simulink model "Organic_AH2"  (R2019b)
settings: Solver=VariableStepAuto  StartTime=0.0  StopTime=t_sim  RelTol=1e-3
InitFcn:
  | clc
  | %clear
  | Ci = 10e-12;
  | t_sim = 40;
  | Vds_max = 10;
  | Vds_min = 0;
  | slope = (Vds_max-Vds_min)/t_sim;
values from neighbouring files (symbols this model uses):
  l = 100e-6    (= 0.0001)    [oAH_main1.m]    (also in oAH_main2.m; oAH_main3.m; oAH_main4.m)
libraries: fl_lib x12, nesl_utility x4
settings Model: Creator=M.J. Mir  LastModifiedBy=yeeyoung
settings SFSimCC: CustomCodeUndefinedFunction=UseInterfaceOnly
settings SimscapeCC: SimscapeNormalizeSystem=off

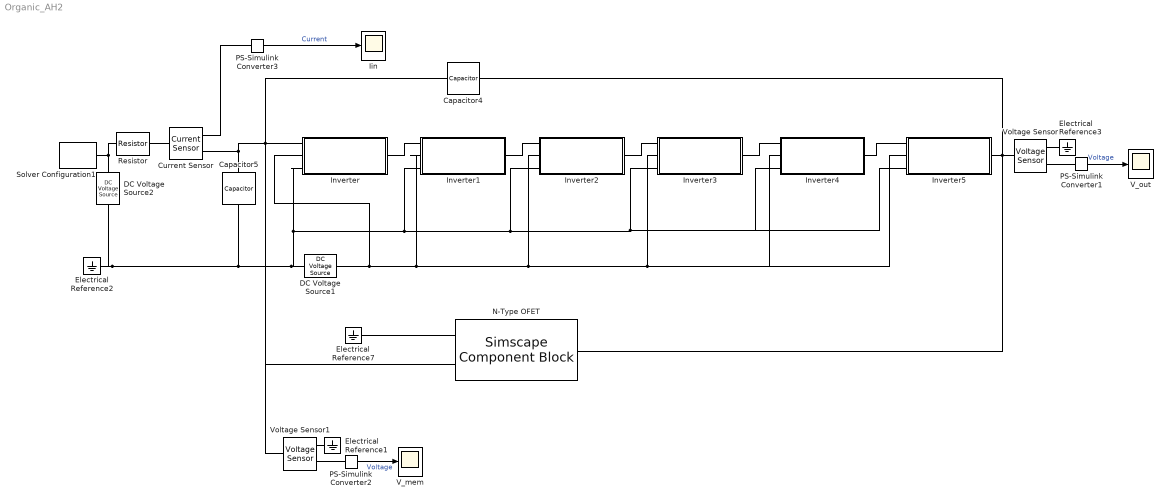
== system Organic_AH2 ==
  Capacitor4 : fl_lib/Electrical/Electrical Elements/Capacitor  c=Cfb nF  r=1e-6 Ohm  g=0 1/Ohm  i_specify=off  i_priority=None  i=0 A  i_nominal_specify=off  i_nominal_unit=A  i_nominal_value=1  v_specify=off  v_priority=None  v=0 V  v_nominal_specify=off  v_nominal_unit=V  v_nominal_value=1  vc_specify=off  vc_priority=High  vc=0 V  vc_nominal_specify=off  vc_nominal_unit=V  vc_nominal_value=1
  Capacitor5 : fl_lib/Electrical/Electrical Elements/Capacitor  c=Cmem nF  r=1e-6 Ohm  g=0 1/Ohm  i_specify=off  i_priority=None  i=0 A  i_nominal_specify=off  i_nominal_unit=A  i_nominal_value=1  v_specify=off  v_priority=None  v=0 V  v_nominal_specify=off  v_nominal_unit=V  v_nominal_value=1  vc_specify=off  vc_priority=High  vc=0 V  vc_nominal_specify=off  vc_nominal_unit=V  vc_nominal_value=1
  Current Sensor : fl_lib/Electrical/Electrical Sensors/Current Sensor
  DC Voltage Source1 : fl_lib/Electrical/Electrical Sources/DC Voltage Source  v0=Vdd V
  DC Voltage Source2 : fl_lib/Electrical/Electrical Sources/DC Voltage Source  v0=Vin V
  Electrical Reference{1..3,7} (4 alike) : fl_lib/Electrical/Electrical Elements/Electrical Reference
  Iin : Scope
  Inverter : Subsystem
  Inverter1 : Subsystem
  Inverter2 : Subsystem
  Inverter3 : Subsystem
  Inverter4 : Subsystem
  Inverter5 : Subsystem
  N-Type OFET : SimscapeComponentBlock  SourceFile=N_Marinov_OFET  ComponentPath=N_Marinov_OFET  ComponentVariants=N_Marinov_OFET  ComponentVariantNames=N_Marinov_OFET  ClassName=N_Marinov_OFET  SchemaVersion=1  Gamma=gama_n  Lambda=landa_n  Vbb=Vbb_n  Vss=Vss_n  Mu0=mu0_n  Vt=Vt_n V  Cox=ci  W=W_n  L=l  i_specify=off  i_priority=None  i=0 A  i_nominal_specify=off  i_nominal_unit=A  i_nominal_value=1  Vgs_specify=off  Vgs_priority=None  Vgs=0 V  Vgs_nominal_specify=off  Vgs_nominal_unit=V  Vgs_nominal_value=1  Vds_specify=off  Vds_priority=None  Vds=0 V  Vds_nominal_specify=off  Vds_nominal_unit=V  Vds_nominal_value=1
      settings: CopyFcn=simscape.engine.sli.internal.componentblockcallback(gcbh,'COPY')  PreCopyFcn=simscape.engine.sli.internal.componentblockcallback(gcbh,'PRECOPY')  PreDeleteFcn=simscape.engine.sli.internal.componentblockcallback(gcbh,'PREDELETE')  InternalSimscapePortConfiguration="{\"Bottom\":[],\"Left\":[{\"id\":\"g\",\"label\":\"Gate\",\"type\":\"foundation.electrical.electrical\"}],\"Right\":[{\"id\":\"d\",\"label\":\"Drain\",\"type\":\"foundation.electrical.electrical\"},{\"id\":\"s\",\"label\":\"Source\",\"type\":\"foundation.electrical.electrical\"}],\"Top\":[]}"
      mask Type: Marinov OFET
  PS-Simulink Converter1 : nesl_utility/PS-Simulink Converter  PhysicalDomain=network_engine_domain  SubClassName=ps_output  LeftPortType=input  RightPortType=output  PseudoPeriodic=off  Frequencies=[]  Unit=1  AffineConversion=off
  PS-Simulink Converter2 : nesl_utility/PS-Simulink Converter  PhysicalDomain=network_engine_domain  SubClassName=ps_output  LeftPortType=input  RightPortType=output  PseudoPeriodic=off  Frequencies=[]  Unit=1  AffineConversion=off
  PS-Simulink Converter3 : nesl_utility/PS-Simulink Converter  PhysicalDomain=network_engine_domain  SubClassName=ps_output  LeftPortType=input  RightPortType=output  PseudoPeriodic=off  Frequencies=[]  Unit=1  AffineConversion=off
  Resistor : fl_lib/Electrical/Electrical Elements/Resistor  R=10 MOhm  i_specify=off  i_priority=None  i=0 A  i_nominal_specify=off  i_nominal_unit=A  i_nominal_value=1  v_specify=off  v_priority=None  v=0 V  v_nominal_specify=off  v_nominal_unit=V  v_nominal_value=1
  Solver Configuration1 : nesl_utility/Solver Configuration  PhysicalDomain=network_engine_domain  SubClassName=solver  LeftPortType=input  RightPortType=generic  Tones=[]  Harmonics=[]  SimulateNoise=off  Profile=off  UseLocalSampling=off  EnableSwitchedLinearOptims=on  FrequencyDomain=off  UseCCode=off  RelTol=0.001  AbsTol=1e-06  MinStep=1e-09  ToWorkspace=off  RevertToSquareIcSolve=off  NumHomotopyIterations=100  PhasorMode=off  PhasorModeNumHarmonics=1  DoDC=off  ResidualTolerance=1e-09  UseLocalSolver=off  LocalSolverChoice=NE_BACKWARD_EULER_ADVANCER  LocalSolverSampleTime=0.001  DoFixedCost=off  MaxNonlinIter=3  MaxModeIter=2  LinearAlgebra=auto  EquationFormulation=NE_TIME_EF  DelaysMemoryBudget=1024  AutomaticFiltering=off  FilteringTimeConstant=0.001  PartitionStorageMethod=AS_NEEDED  PartitionMemoryBudget=1024  PartitionMethod=ROBUST
  V_mem : Scope
  V_out : Scope
  Voltage Sensor : fl_lib/Electrical/Electrical Sensors/Voltage Sensor
  Voltage Sensor1 : fl_lib/Electrical/Electrical Sensors/Voltage Sensor
  wires:
  PS-Simulink Converter1/1 -> V_out/1  "Voltage"
  PS-Simulink Converter2/1 -> V_mem/1  "Voltage"
  PS-Simulink Converter3/1 -> Iin/1  "Current"
  connections:
  Electrical Reference2/LConn1 -- DC Voltage Source2/RConn1 -- Capacitor5/RConn1 -- Inverter1/LConn3 -- Inverter5/LConn3 -- Inverter4/LConn3 -- Inverter3/LConn3 -- Inverter2/LConn3 -- Inverter/LConn3 -- DC Voltage Source1/RConn1
  Voltage Sensor/RConn1 -- PS-Simulink Converter1/LConn1
  Voltage Sensor/RConn2 -- Electrical Reference3/LConn1
  Capacitor5/LConn1 -- Current Sensor/RConn2 -- N-Type OFET/RConn1 -- Voltage Sensor1/LConn1 -- Inverter/LConn1 -- Capacitor4/LConn1
  DC Voltage Source2/LConn1 -- Solver Configuration1/RConn1 -- Resistor/LConn1
  Inverter1/LConn1 -- Inverter/RConn1
  Inverter1/RConn1 -- Inverter2/LConn1
  Inverter2/RConn1 -- Inverter3/LConn1
  Inverter4/LConn2 -- Inverter5/LConn2 -- Inverter3/LConn2 -- Inverter2/LConn2 -- Inverter1/LConn2 -- Inverter/LConn2 -- DC Voltage Source1/LConn1
  Voltage Sensor1/RConn2 -- Electrical Reference1/LConn1
  Voltage Sensor1/RConn1 -- PS-Simulink Converter2/LConn1
  N-Type OFET/RConn2 -- Electrical Reference7/LConn1
  Inverter5/RConn1 -- Voltage Sensor/LConn1 -- N-Type OFET/LConn1 -- Capacitor4/RConn1
  Inverter4/LConn1 -- Inverter3/RConn1
  Inverter5/LConn1 -- Inverter4/RConn1
  Resistor/RConn1 -- Current Sensor/LConn1
  PS-Simulink Converter3/LConn1 -- Current Sensor/RConn1

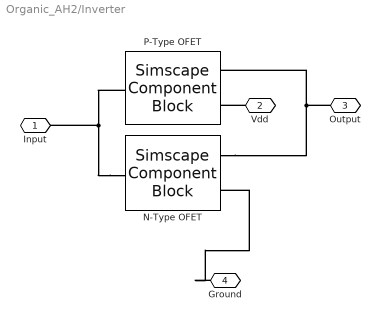
== system Organic_AH2/Inverter ==
  N-Type OFET : SimscapeComponentBlock  SourceFile=N_Marinov_OFET  ComponentPath=N_Marinov_OFET  ComponentVariants=N_Marinov_OFET  ComponentVariantNames=N_Marinov_OFET  ClassName=N_Marinov_OFET  SchemaVersion=1  Gamma=gama_n  Lambda=landa_n  Vbb=Vbb_n  Vss=Vss_n  Mu0=mu0_n  Vt=Vt_n V  Cox=ci  W=W_n  L=l  i_specify=off  i_priority=None  i=0 A  i_nominal_specify=off  i_nominal_unit=A  i_nominal_value=1  Vgs_specify=off  Vgs_priority=None  Vgs=0 V  Vgs_nominal_specify=off  Vgs_nominal_unit=V  Vgs_nominal_value=1  Vds_specify=off  Vds_priority=None  Vds=0 V  Vds_nominal_specify=off  Vds_nominal_unit=V  Vds_nominal_value=1
      settings: CopyFcn=simscape.engine.sli.internal.componentblockcallback(gcbh,'COPY')  PreCopyFcn=simscape.engine.sli.internal.componentblockcallback(gcbh,'PRECOPY')  PreDeleteFcn=simscape.engine.sli.internal.componentblockcallback(gcbh,'PREDELETE')  InternalSimscapePortConfiguration="{\"Bottom\":[],\"Left\":[{\"id\":\"g\",\"label\":\"Gate\",\"type\":\"foundation.electrical.electrical\"}],\"Right\":[{\"id\":\"d\",\"label\":\"Drain\",\"type\":\"foundation.electrical.electrical\"},{\"id\":\"s\",\"label\":\"Source\",\"type\":\"foundation.electrical.electrical\"}],\"Top\":[]}"
      mask Type: Marinov OFET
  P-Type OFET : SimscapeComponentBlock  SourceFile=P_Marinov_OFET  ComponentPath=P_Marinov_OFET  ComponentVariants=P_Marinov_OFET  ComponentVariantNames=P_Marinov_OFET  ClassName=P_Marinov_OFET  SchemaVersion=1  Gamma=gama_p  Lambda=landa_p  Vbb=Vbb_p  Vss=Vss_p  Mu0=mu0_p  Vt=Vt_p V  Cox=ci  W=W_p  L=l  i_specify=off  i_priority=None  i=0 A  i_nominal_specify=off  i_nominal_unit=A  i_nominal_value=1  Vsg_specify=off  Vsg_priority=None  Vsg=0 V  Vsg_nominal_specify=off  Vsg_nominal_unit=V  Vsg_nominal_value=1  Vsd_specify=off  Vsd_priority=None  Vsd=0 V  Vsd_nominal_specify=off  Vsd_nominal_unit=V  Vsd_nominal_value=1
      settings: CopyFcn=simscape.engine.sli.internal.componentblockcallback(gcbh,'COPY')  PreCopyFcn=simscape.engine.sli.internal.componentblockcallback(gcbh,'PRECOPY')  PreDeleteFcn=simscape.engine.sli.internal.componentblockcallback(gcbh,'PREDELETE')  InternalSimscapePortConfiguration="{\"Bottom\":[],\"Left\":[{\"id\":\"g\",\"label\":\"Gate\",\"type\":\"foundation.electrical.electrical\"}],\"Right\":[{\"id\":\"s\",\"label\":\"Source\",\"type\":\"foundation.electrical.electrical\"},{\"id\":\"d\",\"label\":\"Drain\",\"type\":\"foundation.electrical.electrical\"}],\"Top\":[]}"
      mask Type: Marinov OFET
  Input : PMIOPort  Side=Left
  Vdd : PMIOPort  Port=2  Side=Left
  Output : PMIOPort  Port=3  Side=Right
  Ground : PMIOPort  Port=4  Side=Left
  connections:
  N-Type OFET/RConn1 -- Output/RConn1 -- P-Type OFET/RConn2
  N-Type OFET/LConn1 -- Input/RConn1 -- P-Type OFET/LConn1
  Ground/RConn1 -- N-Type OFET/RConn2
  Vdd/RConn1 -- P-Type OFET/RConn1

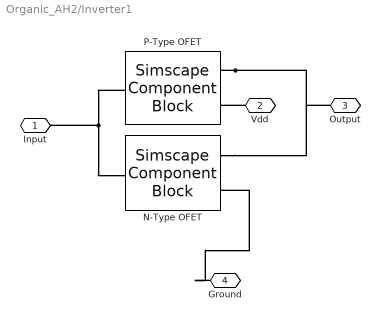
== system Organic_AH2/Inverter1 ==
  N-Type OFET : SimscapeComponentBlock  SourceFile=N_Marinov_OFET  ComponentPath=N_Marinov_OFET  ComponentVariants=N_Marinov_OFET  ComponentVariantNames=N_Marinov_OFET  ClassName=N_Marinov_OFET  SchemaVersion=1  Gamma=gama_n  Lambda=landa_n  Vbb=Vbb_n  Vss=Vss_n  Mu0=mu0_n  Vt=Vt_n V  Cox=ci  W=W_n  L=l  i_specify=off  i_priority=None  i=0 A  i_nominal_specify=off  i_nominal_unit=A  i_nominal_value=1  Vgs_specify=off  Vgs_priority=None  Vgs=0 V  Vgs_nominal_specify=off  Vgs_nominal_unit=V  Vgs_nominal_value=1  Vds_specify=off  Vds_priority=None  Vds=0 V  Vds_nominal_specify=off  Vds_nominal_unit=V  Vds_nominal_value=1
      settings: CopyFcn=simscape.engine.sli.internal.componentblockcallback(gcbh,'COPY')  PreCopyFcn=simscape.engine.sli.internal.componentblockcallback(gcbh,'PRECOPY')  PreDeleteFcn=simscape.engine.sli.internal.componentblockcallback(gcbh,'PREDELETE')  InternalSimscapePortConfiguration="{\"Bottom\":[],\"Left\":[{\"id\":\"g\",\"label\":\"Gate\",\"type\":\"foundation.electrical.electrical\"}],\"Right\":[{\"id\":\"d\",\"label\":\"Drain\",\"type\":\"foundation.electrical.electrical\"},{\"id\":\"s\",\"label\":\"Source\",\"type\":\"foundation.electrical.electrical\"}],\"Top\":[]}"
      mask Type: Marinov OFET
  P-Type OFET : SimscapeComponentBlock  SourceFile=P_Marinov_OFET  ComponentPath=P_Marinov_OFET  ComponentVariants=P_Marinov_OFET  ComponentVariantNames=P_Marinov_OFET  ClassName=P_Marinov_OFET  SchemaVersion=1  Gamma=gama_p  Lambda=landa_p  Vbb=Vbb_p  Vss=Vss_p  Mu0=mu0_p  Vt=Vt_p V  Cox=ci  W=W_p  L=l  i_specify=off  i_priority=None  i=0 A  i_nominal_specify=off  i_nominal_unit=A  i_nominal_value=1  Vsg_specify=off  Vsg_priority=None  Vsg=0 V  Vsg_nominal_specify=off  Vsg_nominal_unit=V  Vsg_nominal_value=1  Vsd_specify=off  Vsd_priority=None  Vsd=0 V  Vsd_nominal_specify=off  Vsd_nominal_unit=V  Vsd_nominal_value=1
      settings: CopyFcn=simscape.engine.sli.internal.componentblockcallback(gcbh,'COPY')  PreCopyFcn=simscape.engine.sli.internal.componentblockcallback(gcbh,'PRECOPY')  PreDeleteFcn=simscape.engine.sli.internal.componentblockcallback(gcbh,'PREDELETE')  InternalSimscapePortConfiguration="{\"Bottom\":[],\"Left\":[{\"id\":\"g\",\"label\":\"Gate\",\"type\":\"foundation.electrical.electrical\"}],\"Right\":[{\"id\":\"s\",\"label\":\"Source\",\"type\":\"foundation.electrical.electrical\"},{\"id\":\"d\",\"label\":\"Drain\",\"type\":\"foundation.electrical.electrical\"}],\"Top\":[]}"
      mask Type: Marinov OFET
  Input : PMIOPort  Side=Left
  Vdd : PMIOPort  Port=2  Side=Left
  Output : PMIOPort  Port=3  Side=Right
  Ground : PMIOPort  Port=4  Side=Left
  connections:
  Vdd/RConn1 -- P-Type OFET/RConn1
  Ground/RConn1 -- N-Type OFET/RConn2
  P-Type OFET/LConn1 -- Input/RConn1 -- N-Type OFET/LConn1
  P-Type OFET/RConn2 -- Output/RConn1 -- N-Type OFET/RConn1

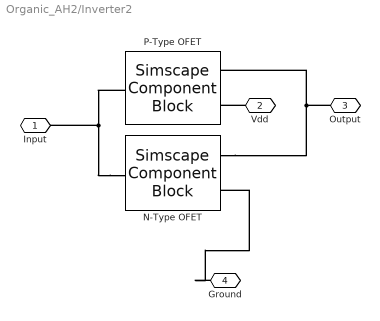
== system Organic_AH2/Inverter2 ==
  N-Type OFET : SimscapeComponentBlock  SourceFile=N_Marinov_OFET  ComponentPath=N_Marinov_OFET  ComponentVariants=N_Marinov_OFET  ComponentVariantNames=N_Marinov_OFET  ClassName=N_Marinov_OFET  SchemaVersion=1  Gamma=gama_n  Lambda=landa_n  Vbb=Vbb_n  Vss=Vss_n  Mu0=mu0_n  Vt=Vt_n V  Cox=ci  W=W_n  L=l  i_specify=off  i_priority=None  i=0 A  i_nominal_specify=off  i_nominal_unit=A  i_nominal_value=1  Vgs_specify=off  Vgs_priority=None  Vgs=0 V  Vgs_nominal_specify=off  Vgs_nominal_unit=V  Vgs_nominal_value=1  Vds_specify=off  Vds_priority=None  Vds=0 V  Vds_nominal_specify=off  Vds_nominal_unit=V  Vds_nominal_value=1
      settings: CopyFcn=simscape.engine.sli.internal.componentblockcallback(gcbh,'COPY')  PreCopyFcn=simscape.engine.sli.internal.componentblockcallback(gcbh,'PRECOPY')  PreDeleteFcn=simscape.engine.sli.internal.componentblockcallback(gcbh,'PREDELETE')  InternalSimscapePortConfiguration="{\"Bottom\":[],\"Left\":[{\"id\":\"g\",\"label\":\"Gate\",\"type\":\"foundation.electrical.electrical\"}],\"Right\":[{\"id\":\"d\",\"label\":\"Drain\",\"type\":\"foundation.electrical.electrical\"},{\"id\":\"s\",\"label\":\"Source\",\"type\":\"foundation.electrical.electrical\"}],\"Top\":[]}"
      mask Type: Marinov OFET
  P-Type OFET : SimscapeComponentBlock  SourceFile=P_Marinov_OFET  ComponentPath=P_Marinov_OFET  ComponentVariants=P_Marinov_OFET  ComponentVariantNames=P_Marinov_OFET  ClassName=P_Marinov_OFET  SchemaVersion=1  Gamma=gama_p  Lambda=landa_p  Vbb=Vbb_p  Vss=Vss_p  Mu0=mu0_p  Vt=Vt_p V  Cox=ci  W=W_p  L=l  i_specify=off  i_priority=None  i=0 A  i_nominal_specify=off  i_nominal_unit=A  i_nominal_value=1  Vsg_specify=off  Vsg_priority=None  Vsg=0 V  Vsg_nominal_specify=off  Vsg_nominal_unit=V  Vsg_nominal_value=1  Vsd_specify=off  Vsd_priority=None  Vsd=0 V  Vsd_nominal_specify=off  Vsd_nominal_unit=V  Vsd_nominal_value=1
      settings: CopyFcn=simscape.engine.sli.internal.componentblockcallback(gcbh,'COPY')  PreCopyFcn=simscape.engine.sli.internal.componentblockcallback(gcbh,'PRECOPY')  PreDeleteFcn=simscape.engine.sli.internal.componentblockcallback(gcbh,'PREDELETE')  InternalSimscapePortConfiguration="{\"Bottom\":[],\"Left\":[{\"id\":\"g\",\"label\":\"Gate\",\"type\":\"foundation.electrical.electrical\"}],\"Right\":[{\"id\":\"s\",\"label\":\"Source\",\"type\":\"foundation.electrical.electrical\"},{\"id\":\"d\",\"label\":\"Drain\",\"type\":\"foundation.electrical.electrical\"}],\"Top\":[]}"
      mask Type: Marinov OFET
  Input : PMIOPort  Side=Left
  Vdd : PMIOPort  Port=2  Side=Left
  Output : PMIOPort  Port=3  Side=Right
  Ground : PMIOPort  Port=4  Side=Left
  connections:
  N-Type OFET/RConn1 -- Output/RConn1 -- P-Type OFET/RConn2
  N-Type OFET/LConn1 -- Input/RConn1 -- P-Type OFET/LConn1
  Ground/RConn1 -- N-Type OFET/RConn2
  Vdd/RConn1 -- P-Type OFET/RConn1

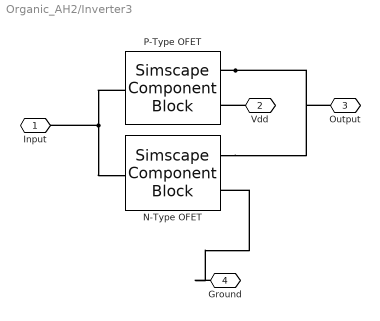
== system Organic_AH2/Inverter3 ==
  N-Type OFET : SimscapeComponentBlock  SourceFile=N_Marinov_OFET  ComponentPath=N_Marinov_OFET  ComponentVariants=N_Marinov_OFET  ComponentVariantNames=N_Marinov_OFET  ClassName=N_Marinov_OFET  SchemaVersion=1  Gamma=gama_n  Lambda=landa_n  Vbb=Vbb_n  Vss=Vss_n  Mu0=mu0_n  Vt=Vt_n V  Cox=ci  W=W_n  L=l  i_specify=off  i_priority=None  i=0 A  i_nominal_specify=off  i_nominal_unit=A  i_nominal_value=1  Vgs_specify=off  Vgs_priority=None  Vgs=0 V  Vgs_nominal_specify=off  Vgs_nominal_unit=V  Vgs_nominal_value=1  Vds_specify=off  Vds_priority=None  Vds=0 V  Vds_nominal_specify=off  Vds_nominal_unit=V  Vds_nominal_value=1
      settings: CopyFcn=simscape.engine.sli.internal.componentblockcallback(gcbh,'COPY')  PreCopyFcn=simscape.engine.sli.internal.componentblockcallback(gcbh,'PRECOPY')  PreDeleteFcn=simscape.engine.sli.internal.componentblockcallback(gcbh,'PREDELETE')  InternalSimscapePortConfiguration="{\"Bottom\":[],\"Left\":[{\"id\":\"g\",\"label\":\"Gate\",\"type\":\"foundation.electrical.electrical\"}],\"Right\":[{\"id\":\"d\",\"label\":\"Drain\",\"type\":\"foundation.electrical.electrical\"},{\"id\":\"s\",\"label\":\"Source\",\"type\":\"foundation.electrical.electrical\"}],\"Top\":[]}"
      mask Type: Marinov OFET
  P-Type OFET : SimscapeComponentBlock  SourceFile=P_Marinov_OFET  ComponentPath=P_Marinov_OFET  ComponentVariants=P_Marinov_OFET  ComponentVariantNames=P_Marinov_OFET  ClassName=P_Marinov_OFET  SchemaVersion=1  Gamma=gama_p  Lambda=landa_p  Vbb=Vbb_p  Vss=Vss_p  Mu0=mu0_p  Vt=Vt_p V  Cox=ci  W=W_p  L=l  i_specify=off  i_priority=None  i=0 A  i_nominal_specify=off  i_nominal_unit=A  i_nominal_value=1  Vsg_specify=off  Vsg_priority=None  Vsg=0 V  Vsg_nominal_specify=off  Vsg_nominal_unit=V  Vsg_nominal_value=1  Vsd_specify=off  Vsd_priority=None  Vsd=0 V  Vsd_nominal_specify=off  Vsd_nominal_unit=V  Vsd_nominal_value=1
      settings: CopyFcn=simscape.engine.sli.internal.componentblockcallback(gcbh,'COPY')  PreCopyFcn=simscape.engine.sli.internal.componentblockcallback(gcbh,'PRECOPY')  PreDeleteFcn=simscape.engine.sli.internal.componentblockcallback(gcbh,'PREDELETE')  InternalSimscapePortConfiguration="{\"Bottom\":[],\"Left\":[{\"id\":\"g\",\"label\":\"Gate\",\"type\":\"foundation.electrical.electrical\"}],\"Right\":[{\"id\":\"s\",\"label\":\"Source\",\"type\":\"foundation.electrical.electrical\"},{\"id\":\"d\",\"label\":\"Drain\",\"type\":\"foundation.electrical.electrical\"}],\"Top\":[]}"
      mask Type: Marinov OFET
  Input : PMIOPort  Side=Left
  Vdd : PMIOPort  Port=2  Side=Left
  Output : PMIOPort  Port=3  Side=Right
  Ground : PMIOPort  Port=4  Side=Left
  connections:
  Vdd/RConn1 -- P-Type OFET/RConn1
  Ground/RConn1 -- N-Type OFET/RConn2
  P-Type OFET/LConn1 -- Input/RConn1 -- N-Type OFET/LConn1
  P-Type OFET/RConn2 -- Output/RConn1 -- N-Type OFET/RConn1

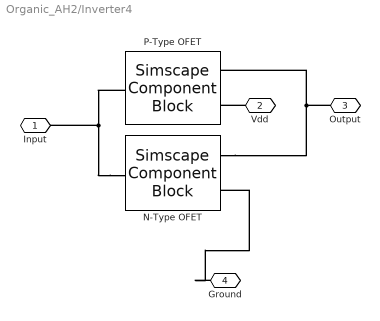
== system Organic_AH2/Inverter4 ==
  N-Type OFET : SimscapeComponentBlock  SourceFile=N_Marinov_OFET  ComponentPath=N_Marinov_OFET  ComponentVariants=N_Marinov_OFET  ComponentVariantNames=N_Marinov_OFET  ClassName=N_Marinov_OFET  SchemaVersion=1  Gamma=gama_n  Lambda=landa_n  Vbb=Vbb_n  Vss=Vss_n  Mu0=mu0_n  Vt=Vt_n V  Cox=ci  W=W_n  L=l  i_specify=off  i_priority=None  i=0 A  i_nominal_specify=off  i_nominal_unit=A  i_nominal_value=1  Vgs_specify=off  Vgs_priority=None  Vgs=0 V  Vgs_nominal_specify=off  Vgs_nominal_unit=V  Vgs_nominal_value=1  Vds_specify=off  Vds_priority=None  Vds=0 V  Vds_nominal_specify=off  Vds_nominal_unit=V  Vds_nominal_value=1
      settings: CopyFcn=simscape.engine.sli.internal.componentblockcallback(gcbh,'COPY')  PreCopyFcn=simscape.engine.sli.internal.componentblockcallback(gcbh,'PRECOPY')  PreDeleteFcn=simscape.engine.sli.internal.componentblockcallback(gcbh,'PREDELETE')  InternalSimscapePortConfiguration="{\"Bottom\":[],\"Left\":[{\"id\":\"g\",\"label\":\"Gate\",\"type\":\"foundation.electrical.electrical\"}],\"Right\":[{\"id\":\"d\",\"label\":\"Drain\",\"type\":\"foundation.electrical.electrical\"},{\"id\":\"s\",\"label\":\"Source\",\"type\":\"foundation.electrical.electrical\"}],\"Top\":[]}"
      mask Type: Marinov OFET
  P-Type OFET : SimscapeComponentBlock  SourceFile=P_Marinov_OFET  ComponentPath=P_Marinov_OFET  ComponentVariants=P_Marinov_OFET  ComponentVariantNames=P_Marinov_OFET  ClassName=P_Marinov_OFET  SchemaVersion=1  Gamma=gama_p  Lambda=landa_p  Vbb=Vbb_p  Vss=Vss_p  Mu0=mu0_p  Vt=Vt_p V  Cox=ci  W=W_p  L=l  i_specify=off  i_priority=None  i=0 A  i_nominal_specify=off  i_nominal_unit=A  i_nominal_value=1  Vsg_specify=off  Vsg_priority=None  Vsg=0 V  Vsg_nominal_specify=off  Vsg_nominal_unit=V  Vsg_nominal_value=1  Vsd_specify=off  Vsd_priority=None  Vsd=0 V  Vsd_nominal_specify=off  Vsd_nominal_unit=V  Vsd_nominal_value=1
      settings: CopyFcn=simscape.engine.sli.internal.componentblockcallback(gcbh,'COPY')  PreCopyFcn=simscape.engine.sli.internal.componentblockcallback(gcbh,'PRECOPY')  PreDeleteFcn=simscape.engine.sli.internal.componentblockcallback(gcbh,'PREDELETE')  InternalSimscapePortConfiguration="{\"Bottom\":[],\"Left\":[{\"id\":\"g\",\"label\":\"Gate\",\"type\":\"foundation.electrical.electrical\"}],\"Right\":[{\"id\":\"s\",\"label\":\"Source\",\"type\":\"foundation.electrical.electrical\"},{\"id\":\"d\",\"label\":\"Drain\",\"type\":\"foundation.electrical.electrical\"}],\"Top\":[]}"
      mask Type: Marinov OFET
  Input : PMIOPort  Side=Left
  Vdd : PMIOPort  Port=2  Side=Left
  Output : PMIOPort  Port=3  Side=Right
  Ground : PMIOPort  Port=4  Side=Left
  connections:
  N-Type OFET/RConn1 -- Output/RConn1 -- P-Type OFET/RConn2
  N-Type OFET/LConn1 -- Input/RConn1 -- P-Type OFET/LConn1
  Ground/RConn1 -- N-Type OFET/RConn2
  Vdd/RConn1 -- P-Type OFET/RConn1

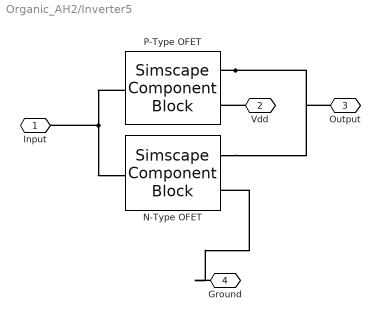
== system Organic_AH2/Inverter5 ==
  N-Type OFET : SimscapeComponentBlock  SourceFile=N_Marinov_OFET  ComponentPath=N_Marinov_OFET  ComponentVariants=N_Marinov_OFET  ComponentVariantNames=N_Marinov_OFET  ClassName=N_Marinov_OFET  SchemaVersion=1  Gamma=gama_n  Lambda=landa_n  Vbb=Vbb_n  Vss=Vss_n  Mu0=mu0_n  Vt=Vt_n V  Cox=ci  W=W_n  L=l  i_specify=off  i_priority=None  i=0 A  i_nominal_specify=off  i_nominal_unit=A  i_nominal_value=1  Vgs_specify=off  Vgs_priority=None  Vgs=0 V  Vgs_nominal_specify=off  Vgs_nominal_unit=V  Vgs_nominal_value=1  Vds_specify=off  Vds_priority=None  Vds=0 V  Vds_nominal_specify=off  Vds_nominal_unit=V  Vds_nominal_value=1
      settings: CopyFcn=simscape.engine.sli.internal.componentblockcallback(gcbh,'COPY')  PreCopyFcn=simscape.engine.sli.internal.componentblockcallback(gcbh,'PRECOPY')  PreDeleteFcn=simscape.engine.sli.internal.componentblockcallback(gcbh,'PREDELETE')  InternalSimscapePortConfiguration="{\"Bottom\":[],\"Left\":[{\"id\":\"g\",\"label\":\"Gate\",\"type\":\"foundation.electrical.electrical\"}],\"Right\":[{\"id\":\"d\",\"label\":\"Drain\",\"type\":\"foundation.electrical.electrical\"},{\"id\":\"s\",\"label\":\"Source\",\"type\":\"foundation.electrical.electrical\"}],\"Top\":[]}"
      mask Type: Marinov OFET
  P-Type OFET : SimscapeComponentBlock  SourceFile=P_Marinov_OFET  ComponentPath=P_Marinov_OFET  ComponentVariants=P_Marinov_OFET  ComponentVariantNames=P_Marinov_OFET  ClassName=P_Marinov_OFET  SchemaVersion=1  Gamma=gama_p  Lambda=landa_p  Vbb=Vbb_p  Vss=Vss_p  Mu0=mu0_p  Vt=Vt_p V  Cox=ci  W=W_p  L=l  i_specify=off  i_priority=None  i=0 A  i_nominal_specify=off  i_nominal_unit=A  i_nominal_value=1  Vsg_specify=off  Vsg_priority=None  Vsg=0 V  Vsg_nominal_specify=off  Vsg_nominal_unit=V  Vsg_nominal_value=1  Vsd_specify=off  Vsd_priority=None  Vsd=0 V  Vsd_nominal_specify=off  Vsd_nominal_unit=V  Vsd_nominal_value=1
      settings: CopyFcn=simscape.engine.sli.internal.componentblockcallback(gcbh,'COPY')  PreCopyFcn=simscape.engine.sli.internal.componentblockcallback(gcbh,'PRECOPY')  PreDeleteFcn=simscape.engine.sli.internal.componentblockcallback(gcbh,'PREDELETE')  InternalSimscapePortConfiguration="{\"Bottom\":[],\"Left\":[{\"id\":\"g\",\"label\":\"Gate\",\"type\":\"foundation.electrical.electrical\"}],\"Right\":[{\"id\":\"s\",\"label\":\"Source\",\"type\":\"foundation.electrical.electrical\"},{\"id\":\"d\",\"label\":\"Drain\",\"type\":\"foundation.electrical.electrical\"}],\"Top\":[]}"
      mask Type: Marinov OFET
  Input : PMIOPort  Side=Left
  Vdd : PMIOPort  Port=2  Side=Left
  Output : PMIOPort  Port=3  Side=Right
  Ground : PMIOPort  Port=4  Side=Left
  connections:
  Vdd/RConn1 -- P-Type OFET/RConn1
  Ground/RConn1 -- N-Type OFET/RConn2
  P-Type OFET/LConn1 -- Input/RConn1 -- N-Type OFET/LConn1
  P-Type OFET/RConn2 -- Output/RConn1 -- N-Type OFET/RConn1
